simulink model "DysfunctionsblkBW"  (Simulink 6.3)
settings: Solver=ode45  SolverMode=SingleTasking  StartTime=0.0  StopTime=999999  MaxStep=10  RelTol=1e-3  AbsTol=1e-3
undefined symbols (not defined in the file): k, TI
settings Model: Creator=lfd  LastModifiedBy=lfd  ExtModeAutoUpdateStatusClock=off  StrictBusMsg=None
settings DataIOCC: LimitDataPoints=off  SaveOutput=off  SaveTime=off
settings OptimizationCC: BlockReduction=off  BooleanDataType=off
settings DebuggingCC: SolverPrmCheckMsg=none
settings HardwareCC: TargetUnknown=on
settings STFCustomTargetCC: TargetFcnLib=ansi_tfl_tmw.mat  GenFloatMathFcnCalls=ANSI_C  ModelReferenceCompliant=off  SystemTargetFile=grt.tlc

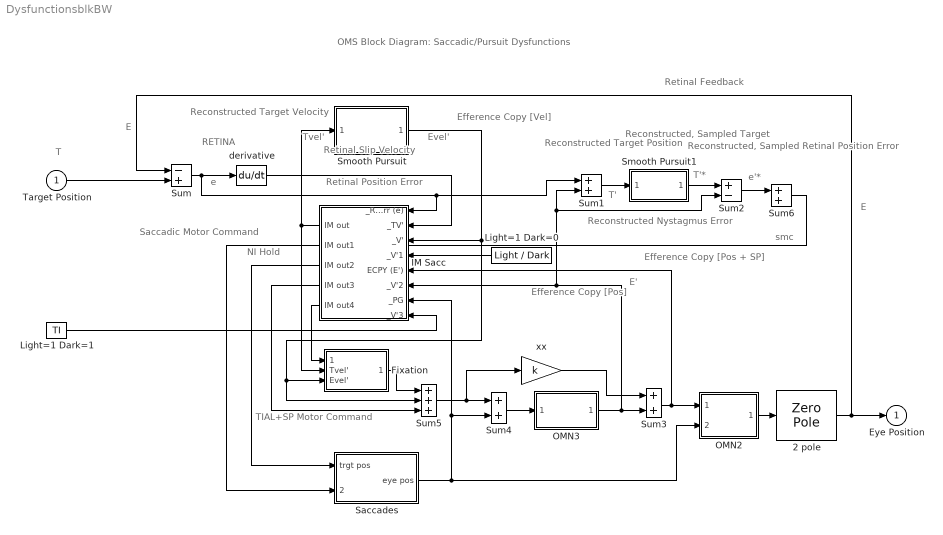
== system DysfunctionsblkBW ==
  note: OMS Block Diagram: Saccadic/Pursuit Dysfunctions
  note: TIAL+SP
      | Motor Command
  note: NI Hold
  note: Saccadic Motor
      | Command
  note: Efference Copy
      | [Vel]
  note: Reconstructed
      | Target Velocity
  note: Efference Copy
      | [Pos]
  note: Efference Copy
      | [Pos + SP]
  note: Retinal Position Error
  note: E
  note: e
  note: E
  note: T
  note: Retinal Feedback
  note: Evel'
  note: E'
  note: Tvel'
  note: Retinal Slip Velocity
  note: RETINA
  note: Reconstructed, Sampled
      | Retinal Position Error
  note: Reconstructed
      | Target Position
  note: T'
  note: e'*
  note: smc
  note: T'*
  note: Reconstructed,
      | Sampled
      | Target
  note: Reconstructed Nystagmus Error
  Target Position : Inport
  2 pole : ZeroPole  Zeros=[ ]  Poles=[ -1/.18 -1/.007]  Gain=[1/.18 * 1/.007]
      mask Display: disp('EOM\n[2-Pole\nPlant]')
  Fixation : Subsystem
      mask Display: disp('Fixation')
  IM Sacc : Subsystem  Orientation=left
      mask Display: disp('INTERNAL\nMONITOR\n[Sacc,FS/BS,\nSP,AL,\nNI Control]')
  Light=1 Dark=0 : Constant  Orientation=left  Value=Light / Dark
  Light=1 Dark=1 : Constant  Value=TI
  OMN2 : Subsystem
      mask Display: disp('OMN\n[Tonic +\nPhasic]')
  OMN3 : Subsystem
      mask Display: disp('Neural \nIntegrator')
  Saccades : Subsystem
      mask Display: disp('Saccadic\n[PG,NI Hold]')
  Smooth Pursuit : Subsystem
      mask Display: disp('Smooth\nPursuit')
  Smooth Pursuit1 : Subsystem
      mask Display: disp('Saccadic\nSampler')
  Sum : Sum  Inputs=-+  SaturateOnIntegerOverflow=on  InputSameDT=on
  Sum{1,3..4,6} (4 alike) : Sum  SaturateOnIntegerOverflow=on  InputSameDT=on
  Sum2 : Sum  Inputs=+-  SaturateOnIntegerOverflow=on  InputSameDT=on
  Sum5 : Sum  Inputs=+++  SaturateOnIntegerOverflow=on  InputSameDT=on
  derivative : Derivative
      mask Display: disp('s')
  xx : Gain  Gain=k  SaturateOnIntegerOverflow=on
  Eye Position : Outport  InitialOutput=0
  wires:
  derivative/1 -> IM Sacc/2(_TV')
  Sum/1 -> derivative/1, IM Sacc/1(_RetErr (e)), Sum1/1
  Light=1 Dark=0/1 -> IM Sacc/4(_V'1)
  xx/1 -> Sum3/1
  IM Sacc/2(IM out1) -> Saccades/2()
  IM Sacc/3(IM out2) -> Saccades/1(trgt pos)
  Saccades/1(eye pos) -> Sum4/2, IM Sacc/7(_PG), OMN2/2(from PG)
  Light=1 Dark=1/1 -> IM Sacc/8(_V'3)
  OMN3/1(out_1) -> Sum3/2, IM Sacc/6(_V'2), Sum1/2, Sum2/2
  Sum3/1 -> IM Sacc/5(ECPY (E')), OMN2/1(from NI)
  OMN2/1(out_1) -> 2 pole/1
  Sum4/1 -> OMN3/1(from NI)
  Smooth Pursuit/1(eye pos) -> IM Sacc/3(_V'), Fixation/3(Evel'), Sum5/2
  IM Sacc/5(IM out4) -> Fixation/1(fs [fsmc30])
  IM Sacc/1(IM out) -> Smooth Pursuit/1(trgt pos), Fixation/2(Tvel')
  IM Sacc/4(IM out3) -> Sum5/3
  Fixation/1(" CorrVel [velcorr]") -> Sum5/1
  Sum5/1 -> Sum4/1, xx/1
  2 pole/1 -> Eye Position/1, Sum/1
  Target Position/1 -> Sum/2
  Sum6/1 -> ?
  ? -> Sum6/2
  Sum1/1 -> Smooth Pursuit1/1(trgt pos)
  Smooth Pursuit1/1(eye pos) -> Sum2/1
  Sum2/1 -> Sum6/1

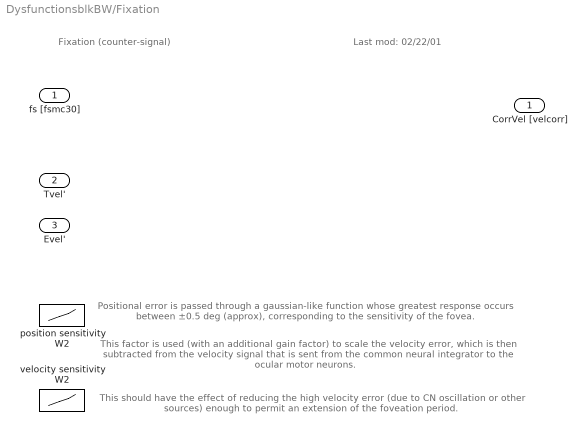
== system DysfunctionsblkBW/Fixation ==
  note: Fixation (counter-signal)
  note: Last mod: 02/22/01
  note: Positional error is passed through a gaussian-like function whose greatest
      | response occurs between ±0.5 deg (approx), corresponding to the sensitivity
      | of the fovea.
  note: This factor is used (with an additional gain factor) to scale the velocity error,
      | which is then subtracted from the velocity signal that is sent from the
      | common neural integrator to the ocular motor neurons.
  note: This should have the effect of reducing the high velocity error (due
      | to CN oscillation or other sources) enough to permit an extension of
      | the foveation period.
  fs [fsmc30] : Inport
  Tvel' : Inport  Port=2
  Evel' : Inport  Port=3
  position sensitivity W2 : Lookup  InputValues="[-5 -2  -1 -0.5   0.5   1    2    5]"  OutputValues="[ 0   0.125    0.5     1      1     0.5    0.125  0]"  SaturateOnIntegerOverflow=on
  velocity sensitivity W2 : Lookup  InputValues="[-30 -15   -8  -4   4     8  15  30]"  OutputValues="[0  0.125   0.5    1    1    0.5   0.125  0]"  SaturateOnIntegerOverflow=on
  " CorrVel [velcorr]" : Outport  InitialOutput=0
  wires:
  ? -> " CorrVel [velcorr]"/1

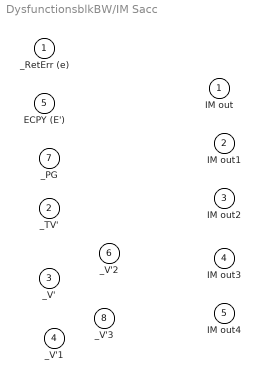
== system DysfunctionsblkBW/IM Sacc ==
  _RetErr (e) : Inport
  _TV' : Inport  Port=2
  _V' : Inport  Port=3
  _V'1 : Inport  Port=4
  ECPY (E') : Inport  Port=5
  _V'2 : Inport  Port=6
  _PG : Inport  Port=7
  _V'3 : Inport  Port=8
  IM out : Outport  InitialOutput=0
  IM out1 : Outport  Port=2  InitialOutput=0
  IM out2 : Outport  Port=3  InitialOutput=0
  IM out3 : Outport  Port=4  InitialOutput=0
  IM out4 : Outport  Port=5  InitialOutput=0

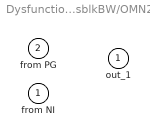
== system DysfunctionsblkBW/OMN2 ==
  from NI : Inport
  from PG : Inport  Port=2
  out_1 : Outport  InitialOutput=0

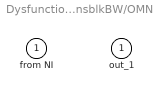
== system DysfunctionsblkBW/OMN3 ==
  from NI : Inport
  out_1 : Outport  InitialOutput=0

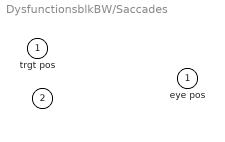
== system DysfunctionsblkBW/Saccades ==
  trgt pos : Inport
   : Inport  Port=2
  eye pos : Outport  InitialOutput=0

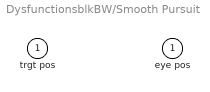
== system DysfunctionsblkBW/Smooth Pursuit ==
  trgt pos : Inport
  eye pos : Outport  InitialOutput=0

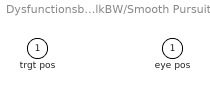
== system DysfunctionsblkBW/Smooth Pursuit1 ==
  trgt pos : Inport
  eye pos : Outport  InitialOutput=0
